simulink model "LoadFlow116BusNetwork_original"  (R2024a)
settings: Solver=FixedStepDiscrete  StartTime=0.0  StopTime=4.5  FixedStep=75e-6  RelTol=1e-3  EnableMultiTasking=on
undefined symbols (not defined in the file or in its folder): D1, D11, Delta
libraries: spsSeriesRLCBranchLib x164, spsLoadFlowBusLib x116, spsDistributedParametersLineLib x79, spsThreePhaseSeriesRLCLoadLib x60, spsThreePhaseTransformerTwoWindingsLib x52, spsThreePhaseParallelRLCLoadLib x44, spsThreePhaseVIMeasurementLib x44, spsSynchronousMachinepuStandardLib x28, spsExcitationSystemLib x28, spsHydraulicTurbineandGovernorLib x28, spsGenericPowerSystemStabilizerLib x28, spsMultiBandPowerSystemStabilizerLib x28
(part 10 of 15)

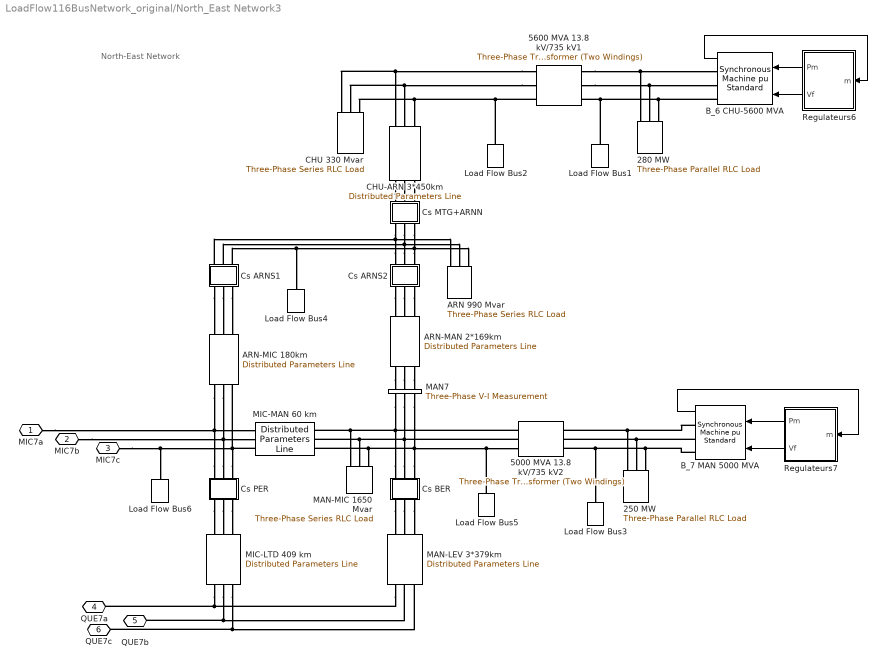
== system LoadFlow116BusNetwork_original/North_East Network3 ==
  note: North-East Network
  250 MW : spsThreePhaseParallelRLCLoadLib/Three-Phase Parallel RLC Load  LConnTagsString=A|B|C  Configuration=Y (grounded)  NominalVoltage=(13800)*1  Vabc=[1e3 1e3 1e3]  Vabcp=[1e3 1e3 1e3]  NominalFrequency=60  UnbalancedPower=off  ActivePower=250000000  InductivePower=0  CapacitivePower=0  Pabc=[10e3 9e3 11e3]  QLabc=[100 90 110]  QCabc=[100 90 110]  Pabcp=[10e3 9e3 11e3]  QLabcp=[100 90 110]  QCabcp=[100 90 110]  Measurements=None  LoadType=constant PQ
  280 MW : spsThreePhaseParallelRLCLoadLib/Three-Phase Parallel RLC Load  LConnTagsString=A|B|C  Configuration=Y (grounded)  NominalVoltage=(13800)*1  Vabc=[1e3 1e3 1e3]  Vabcp=[1e3 1e3 1e3]  NominalFrequency=60  UnbalancedPower=off  ActivePower=280000000  InductivePower=0  CapacitivePower=0  Pabc=[10e3 9e3 11e3]  QLabc=[100 90 110]  QCabc=[100 90 110]  Pabcp=[10e3 9e3 11e3]  QLabcp=[100 90 110]  QCabcp=[100 90 110]  Measurements=None  LoadType=constant PQ
  5000 MVA 13.8 kV/735 kV2 : spsThreePhaseTransformerTwoWindingsLib/Three-Phase Transformer (Two Windings)  Winding1Connection=Delta (D1)  Winding2Connection=Yg  CoreType=Three single-phase transformers  SetSaturation=off  Hysteresis=off  DataFile='basic_model'  SetInitialFlux=off  Measurements=None  UNITS=pu  NominalPower=[ 5000e6 60 ]  Winding1="[ 13.8e3 0.002  0.0]"  Winding2=[ 735e3 0.002 0.12]  Rm=500  Lm=500  L0=0.5  Saturation="[ 0,0  ;  0.005,1.2  ;  1.0,1.4 ]"  InitialFluxes=[ 0.8 , -0.8 , 0.7 ]  BreakLoop=off  DiscreteSolver=Trapezoidal iterative  DataType=off  TransfoNumber=0
  5600 MVA 13.8 kV/735 kV1 : spsThreePhaseTransformerTwoWindingsLib/Three-Phase Transformer (Two Windings)  Winding1Connection=Delta (D1)  Winding2Connection=Yg  CoreType=Three single-phase transformers  SetSaturation=off  Hysteresis=off  DataFile='basic_model'  SetInitialFlux=off  Measurements=None  UNITS=pu  NominalPower=[ 5600e6 60 ]  Winding1="[ 13.8e3 0.002  0.0]"  Winding2=[ 735e3 0.002 0.12]  Rm=500  Lm=500  L0=0.5  Saturation="[ 0,0  ;  0.005,1.2  ;  1.0,1.4 ]"  InitialFluxes=[ 0.8 , -0.8 , 0.7 ]  BreakLoop=off  DiscreteSolver=Trapezoidal iterative  DataType=off  TransfoNumber=0
  ARN 990 Mvar : spsThreePhaseSeriesRLCLoadLib/Three-Phase Series RLC Load  LConnTagsString=A|B|C  Configuration=Y (grounded)  NominalVoltage=735e3  Vabc=[1e3 1e3 1e3]  Vabcp=[1e3 1e3 1e3]  NominalFrequency=60  UnbalancedPower=off  ActivePower=3300000  InductivePower=990e6  CapacitivePower=0  Pabc=[10e3 9e3 11e3]  QLabc=[100 90 110]  QCabc=[100 90 110]  Pabcp=[10e3 9e3 11e3]  QLabcp=[100 90 110]  QCabcp=[100 90 110]  Measurements=None  LoadType=constant Z
  ARN-MAN 2*169km : spsDistributedParametersLineLib/Distributed Parameters Line  Phases=3  Length=169  Frequency=60  Resistance="[0.01273  0.3864]/2"  Inductance="[0.9337e-3  4.1264e-3]/2"  Capacitance=[12.74e-9 7.751e-9]*2  x1=[-0.000975 6.97288339187692e-10 276427.296115167 -784420.047795391;-0.0009 5.9086446365215e-10 298492.841238258 -776291.834335168;-0.000825 4.83968260104895e-10 320319.775751156 -767543.065060241;-0.00075 3.76685179735474e-10 341890.651536376 -758180.733602908;-0.000675 2.69100982996849e-10 363188.22516586 -748212.324067686;-0.0006 1.613016710498e-10 384195.471685113 -737645.805048638;-0.000525 5.33734170149115e-11 404895.598222688 -726489.623259392;-0.00045 -5.45975029128977e-11 425272.057414155 -714752.696780978;-0.000375 -1.62524778432248e-10 445308.560629805 -702444.407932839;-0.0003 -2.70322134130433e-10 464989.090995538 -689574.595772759;-0.000225 -3.7790339845066e-10 484297.9161965 -676153.548231663;-0.00015 -4.85182572576282e-10 503219.601053261 -662191.993889607;-7.5e-05 -5.9207389917693e-10 521739.019860459 -647701.093399513]  x2=[-0.000975 1.79211182163766e-09 170603.864508898 -782532.609847016;-0.0009 1.69187859903041e-09 192658.333570984 -777396.800423744;-0.000825 1.59029291455771e-09 214558.794508984 -771639.551892782;-0.00075 1.48743597426141e-09 236287.740429513 -765265.466510519;-0.000675 1.38339000040582e-09 257827.801545667 -758279.639623281;-0.0006 1.27823816575047e-09 279161.759062162 -750687.655594196;-0.000525 1.17206452706313e-09 300272.558939782 -742495.583339135;-0.00045 1.06495395792605e-09 321143.325528109 -733709.971475316;-0.000375 9.56992080889336e-10 341757.375055666 -724337.843086439;-0.0003 8.48265199025631e-10 362098.228966668 -714386.69010854;-0.000225 7.38860226940719e-10 382149.627093722 -703864.46734105;-0.00015 6.28864621295331e-10 401895.540655962 -692779.586087855;-7.5e-05 5.1836631089363e-10 421320.185072211 -681140.907433425]  x3=[-0.000975 1.85817274928847e-12 1329.17201367229 -2414.87241463209;-0.0009 1.81508564794597e-12 1396.90953145523 -2376.3316706908;-0.000825 1.77054759490824e-12 1463.53038113216 -2335.89132357105;-0.00075 1.72459419321344e-12 1528.98130701517 -2293.58370066758;-0.000675 1.67726217730775e-12 1593.20998863556 -2249.4426220468;-0.0006 1.6285893836805e-12 1656.16508256796 -2203.50337341158;-0.000525 1.57861472061818e-12 1717.79626347353 -2155.80267789439;-0.00045 1.52737813710182e-12 1778.05426432925 -2106.37866670137;-0.000375 1.47492059087233e-12 1836.8909158112 -2055.27084863088;-0.0003 1.42128401568954e-12 1894.25918480043 -2002.52007849068;-0.000225 1.36651128781098e-12 1950.11321198046 -1948.16852443932;-0.00015 1.31064619171726e-12 2004.40834849657 -1892.25963427751;-7.5e-05 1.25373338511145e-12 2057.10119164737 -1834.83810071659]  x4=[-0.000975 2.61332635721004e-12 681.724417841508 -9455.17189861359;-0.0009 2.14673687942227e-12 948.756484622685 -9432.1197918923;-0.000825 1.67843133301927e-12 1215.03012998652 -9401.52779292565;-0.00075 1.20878407428951e-12 1480.33249885502 -9363.42035648953;-0.000675 7.38170532065782e-13 1744.45151257379 -9317.82794508557;-0.0006 2.66966907613108e-13 2007.17603844441 -9264.78700458986;-0.000525 -2.04450126100782e-13 2268.29605850072 -9204.33993511867;-0.00045 -6.75703725512058e-13 2527.60283739395 -9136.53505713448;-0.000375 -1.14641717770377e-12 2784.8890892526 -9061.42657281928;-0.0003 -1.6162142015444e-12 3039.94914338353 -8979.07452274625;-0.000225 -2.08471924848123e-12 3292.57910868201 -8889.54473788418;-0.00015 -2.55155780274809e-12 3542.57703661917 -8792.90878697324;-7.5e-05 -3.01635668074757e-12 3789.7430826765 -8689.24391931401]  x5=0.000955765248222805  V1=ones(3,3)  V2=ones(3,3)  I1=ones(3,3)  I2=ones(3,3)  nHarmo=1  Measurements=None  Decoupling=off  VsMag0=[ 1 1 1]  VrMag0=[ 1 1 1]  VsAngle0=[0 -120 120]  VrAngle0=[0 -120 120]  IsMag0=[ 1 1 1]  IrMag0=[ 1 1 1]  IsAngle0=[0 -120 120]  IrAngle0=[0 -120 120]
      settings: AttributesFormatString=\n  LibrarySourceBlock=sps_lib/Power Grid Elements/Distributed Parameters Line
  ARN-MIC 180km : spsDistributedParametersLineLib/Distributed Parameters Line  Phases=3  Length=180  Frequency=60  Resistance="[0.01273  0.3864]"  Inductance="[0.9337e-3  4.1264e-3]"  Capacitance=[12.74e-9 7.751e-9]  x1=[-0.00105 9.60262409026762e-10 262529.955827452 -774207.772445399;-0.000975 8.43704923918377e-10 284312.349574713 -766476.523484014;-0.0009 7.26472994002931e-10 305867.468379848 -758132.564917239;-0.000825 6.08660332691488e-10 327178.081410689 -749182.566777887;-0.00075 4.90361117622907e-10 348227.153289243 -739633.683557531;-0.000675 3.71669915379674e-10 368997.857709512 -729493.548487313;-0.0006 2.52681605892828e-10 389473.590888184 -718770.26743606;-0.000525 1.33491306596389e-10 409637.984837447 -707472.412430573;-0.00045 1.41942963919424e-11 429474.920449301 -695609.01480328;-0.000375 -1.0511406051586e-10 448968.540380935 -683189.557972727;-0.0003 -2.24338390851985e-10 468103.261730838 -670223.969862682;-0.000225 -3.43383388510955e-10 486863.788495533 -656722.6149659;-0.00015 -4.62153890743092e-10 505235.12379697 -642696.286058906;-7.5e-05 -5.8055495422616e-10 523202.581870801 -628156.195574421]  x2=[-0.00105 3.56382163731829e-09 126759.491965692 -811882.989724104;-0.000975 3.44933874622974e-09 149661.239004238 -807974.954382786;-0.0009 3.3320985065241e-09 172443.349138217 -803421.036225366;-0.000825 3.21219463825516e-09 195087.610697368 -798224.875584341;-0.00075 3.08972299074063e-09 217575.922205467 -792390.626191025;-0.000675 2.96478146594164e-09 239890.306850379 -785922.951855114;-0.0006 2.83746994020147e-09 262012.926854439 -778827.022736515;-0.000525 2.70789018440583e-09 283926.097733704 -771108.511212393;-0.00045 2.5761457826289e-09 305612.302434655 -762773.587342764;-0.000375 2.44234204932968e-09 327054.205337066 -753828.913938241;-0.0003 2.30658594516532e-09 348234.666111827 -744281.641233884;-0.000225 2.16898599148834e-09 369136.753422667 -734139.401173416;-0.00015 2.02965218359636e-09 389743.758460803 -723410.301308359;-7.5e-05 1.88869590280353e-09 410039.208301705 -712102.918316986]  x3=[-0.00105 4.84689301461233e-12 -44.8517351581199 -825.87934362595;-0.000975 4.94622387761714e-12 -21.4861584034094 -826.817643959817;-0.0009 5.04160080493394e-12 1.89659405757936 -827.094998919837;-0.000825 5.13294755370635e-12 25.2778304102975 -826.711186792699;-0.00075 5.22019110274107e-12 48.6388600521494 -825.666514391943;-0.000675 5.30326171087985e-12 71.9610085334751 -823.961816812704;-0.0006 5.38209297274958e-12 95.2256324856196 -821.598456764144;-0.000525 5.45662187184569e-12 118.414134524156 -818.578323480124;-0.00045 5.52678883090655e-12 141.507978115351 -814.903831208983;-0.000375 5.59253775953869e-12 164.488702393985 -810.57791728362;-0.0003 5.65381609905455e-12 187.337936920687 -805.604039773438;-0.000225 5.71057486448711e-12 210.037416366981 -799.986174720016;-0.00015 5.76276868374773e-12 232.568995116311 -793.728812958723;-7.5e-05 5.81035583389588e-12 254.914661769371 -786.836956528808]  x4=[-0.00105 4.98553141097365e-12 787.856966725554 -5164.02437043783;-0.000975 4.55090288137183e-12 933.53262233862 -5139.68710729464;-0.0009 4.11263642963779e-12 1078.46202625692 -5111.24125691772;-0.000825 3.67108239926734e-12 1222.52932413244 -5078.70955848464;-0.00075 3.22659376179636e-12 1365.61935077159 -5042.11801733737;-0.000675 2.77952583464074e-12 1507.6177221964 -5001.49588419404;-0.0006 2.33023599706108e-12 1648.41092708142 -4956.87563176633;-0.000525 1.87908340447918e-12 1787.88641749285 -4908.29292880132;-0.00045 1.42642870137468e-12 1925.93269885773 -4855.78661156844;-0.000375 9.72633732991387e-13 2062.43941909089 -4799.39865281429;-0.0003 5.18061256083737e-13 2197.29745680882 -4739.17412821035;-0.000225 6.30746489345782e-14 2330.39900855955 -4675.16118032011;-0.00015 -3.91962379123865e-13 2461.63767499914 -4607.41098011468;-7.5e-05 -8.46686078453662e-13 2590.90854594566 -4535.97768606751]  x5=0.00101797482059234  V1=ones(3,3)  V2=ones(3,3)  I1=ones(3,3)  I2=ones(3,3)  nHarmo=1  Measurements=None  Decoupling=off  VsMag0=[ 1 1 1]  VrMag0=[ 1 1 1]  VsAngle0=[0 -120 120]  VrAngle0=[0 -120 120]  IsMag0=[ 1 1 1]  IrMag0=[ 1 1 1]  IsAngle0=[0 -120 120]  IrAngle0=[0 -120 120]
      settings: AttributesFormatString=\n  LibrarySourceBlock=sps_lib/Power Grid Elements/Distributed Parameters Line
  "B_6 CHU-5600 MVA " : spsSynchronousMachinepuStandardLib/Synchronous Machine pu Standard  PresetModel=No  MechanicalLoad=Mechanical power Pm  ShowDetailedParameters=on  RotorType=Salient-pole  Units=per unit standard parameters  MeasurementBus=off  NominalParameters="[ 5600E6  13800   60 ]"  Reactances1=[ 31 32 33 34 35 36 37 ]  Reactances2=[ 1.305, 0.296, 0.252, 0.474, 0.243, 0.18 ]  dAxisTimeConstants=Short-circuit  qAxisTimeConstants=Open-circuit  TimeConstants1=[]  TimeConstants2=[]  TimeConstants3=[]  TimeConstants4=[]  TimeConstants5=[ 1.01, 0.053, 0.1 ]  TimeConstants6=[]  TimeConstants7=[]  TimeConstants8=[]  StatorResistance=2.8544e-3  Mechanical="[ 4.0 0  32]"  PolePairs=32  InitialConditions=[0 -61.7964 0.894782 0.894782 0.894782 8.48442 -111.516 128.484 1.31361]  SetSaturation=off  Saturation=[0.6404,0.7127,0.8441,0.9214,0.9956,1.082,1.19,1.316,1.457;0.7,0.7698,0.8872,0.9466,0.9969,1.046,1.1,1.151,1.201]  LoadFlowParameters=[1 5000000000 0 0 0]  TsPowergui=0  TsBlock=-1  IterativeModel=Trapezoidal non iterative  IterativeDiscreteModel=Trapezoidal non iterative  BusType=PV  Pref=5000000000  Qref=0  Qmin=-Inf  Qmax=Inf  PLF=0  QLF=0
  B_7 MAN 5000 MVA : spsSynchronousMachinepuStandardLib/Synchronous Machine pu Standard  PresetModel=No  MechanicalLoad=Mechanical power Pm  ShowDetailedParameters=on  RotorType=Salient-pole  Units=per unit standard parameters  MeasurementBus=off  NominalParameters="[ 5000E6  13800   60 ]"  Reactances1=[ 31 32 33 34 35 36 37 ]  Reactances2=[ 1.305, 0.296, 0.252, 0.474, 0.243, 0.18 ]  dAxisTimeConstants=Short-circuit  qAxisTimeConstants=Open-circuit  TimeConstants1=[]  TimeConstants2=[]  TimeConstants3=[]  TimeConstants4=[]  TimeConstants5=[ 1.01, 0.053, 0.1 ]  TimeConstants6=[]  TimeConstants7=[]  TimeConstants8=[]  StatorResistance=2.8544e-3  Mechanical="[ 3.7 0  32]"  PolePairs=32  InitialConditions=[0 -81.9543 0.907703 0.907703 0.907703 -8.76021 -128.76 111.24 1.25655]  SetSaturation=off  Saturation=[0.6404,0.7127,0.8441,0.9214,0.9956,1.082,1.19,1.316,1.457;0.7,0.7698,0.8872,0.9466,0.9969,1.046,1.1,1.151,1.201]  LoadFlowParameters=[1 4500000000 0 0 0]  TsPowergui=0  TsBlock=-1  IterativeModel=Trapezoidal non iterative  IterativeDiscreteModel=Trapezoidal non iterative  BusType=PV  Pref=4500000000  Qref=0  Qmin=-Inf  Qmax=Inf  PLF=0  QLF=0
  CHU 330 Mvar : spsThreePhaseSeriesRLCLoadLib/Three-Phase Series RLC Load  LConnTagsString=A|B|C  Configuration=Y (grounded)  NominalVoltage=735e3  Vabc=[1e3 1e3 1e3]  Vabcp=[1e3 1e3 1e3]  NominalFrequency=60  UnbalancedPower=off  ActivePower=1100000  InductivePower=330e6  CapacitivePower=0  Pabc=[10e3 9e3 11e3]  QLabc=[100 90 110]  QCabc=[100 90 110]  Pabcp=[10e3 9e3 11e3]  QLabcp=[100 90 110]  QCabcp=[100 90 110]  Measurements=None  LoadType=constant Z
  CHU-ARN 3*450km : spsDistributedParametersLineLib/Distributed Parameters Line  Phases=3  Length=450  Frequency=60  Resistance="[0.01273  0.3864]/3"  Inductance="[0.9337e-3  4.1264e-3]/3"  Capacitance=[12.74e-9 7.751e-9]*3  x1=[-0.00255 1.27916652564422e-09 0 0;-0.002475 1.19821918273683e-09 0 0;-0.0024 1.11631400174812e-09 0 0;-0.002325 1.03351645642659e-09 0 0;-0.00225 9.4989273386313e-10 0 0;-0.002175 8.65509681582063e-10 0 0;-0.0021 7.80434754104282e-10 0 0;-0.002025 6.94735959025121e-10 0 0;-0.00195 6.08481802650133e-10 0 0;-0.001875 5.2174123523219e-10 0 0;-0.0018 4.34583595853711e-10 0 0;-0.001725 3.47078556998058e-10 0 0;-0.00165 2.59296068854421e-10 0 0;-0.001575 1.71306303400705e-10 242668.421457094 -732167.508894252;-0.0015 8.31795983091243e-11 263270.288908761 -725014.590467024;-0.001425 -5.01359928065404e-12 283661.702119646 -717282.106469271;-0.00135 -9.32027890758778e-11 303826.360506025 -708976.23813039;-0.001275 -1.81317473987565e-10 323748.144748515 -700103.625034449;-0.0012 -2.69287216484797e-10 343411.129677606 -690671.359812599;-0.001125 -3.57041694901403e-10 362799.597003999 -680686.982473342;-0.00105 -4.44510759650027e-10 381898.047883567 -670158.474375156;-0.000975 -5.31624489298628e-10 400691.215306893 -659094.251846322;-0.0009 -6.18313246464612e-10 419164.076303483 -647503.159457043;-0.000825 -7.04507733481883e-10 437301.863950903 -635394.462949224;-0.00075 -7.90139047796337e-10 455090.079179222 -622777.841829585;-0.000675 -8.75138737045516e-10 472514.502361358 -609663.381632008;-0.0006 -9.59438853778372e-10 489561.20468002 -596061.565855317;-0.000525 -1.04297200977143e-09 506216.559262199 -581983.267582929;-0.00045 -1.12567142989787e-09 522467.252072276 -567439.740791078;-0.000375 -1.20747100550661e-09 538300.292555064 -552442.611352557;-0.0003 -1.28830534726847e-09 553703.024020254 -537003.867743177;-0.000225 -1.36810983744746e-09 568663.133759983 -521135.851458357;-0.00015 -1.44682068155518e-09 583168.662891422 -504851.247147528;-7.5e-05 -1.52437495934716e-09 597208.015916525 -488163.072474212]  x2=[-0.00255 2.8073590882473e-09 0 0;-0.002475 2.72875365746816e-09 0 0;-0.0024 2.64796690276658e-09 0 0;-0.002325 2.56506340383818e-09 0 0;-0.00225 2.48010943247153e-09 0 0;-0.002175 2.39317289957151e-09 0 0;-0.0021 2.30432330087236e-09 0 0;-0.002025 2.21363166138381e-09 0 0;-0.00195 2.12117047861485e-09 0 0;-0.001875 2.02701366462028e-09 0 0;-0.0018 1.93123648691657e-09 0 0;-0.001725 1.83391550831412e-09 0 0;-0.00165 1.73512852571417e-09 0 0;-0.001575 1.63495450791913e-09 -54170.2857366766 -807523.190587066;-0.0015 1.5334735325061e-09 -31319.4766466056 -808731.868853668;-0.001425 1.43076672181411e-09 -8443.63124610734 -809294.059238321;-0.00135 1.32691617809617e-09 14438.9638640172 -809209.312334633;-0.001275 1.22200491788796e-09 37310.0166873523 -808477.695887982;-0.0012 1.11611680564569e-09 60151.24445421 -807099.794741363;-0.001125 1.00933648670615e-09 82944.3882365959 -805076.710367868;-0.00105 9.01749319622503e-10 105671.227544117 -802410.059990191;-0.000975 7.93441307929975e-10 128313.594889164 -799101.975287844;-0.0009 6.84499031395948e-10 150853.39030972 -795155.100693122;-0.000825 5.75009576809409e-10 173272.595838196 -790572.591277188;-0.00075 4.65060468365111e-10 195553.289904719 -785358.110227952;-0.000675 3.54739597698064e-10 217677.661663358 -779515.825921782;-0.0006 2.44135153624316e-10 239628.025229844 -773050.408591363;-0.000525 1.33335551644154e-10 261386.833819392 -765967.026592383;-0.00045 2.24293632641098e-11 282936.693773338 -758271.342272034;-0.000375 -8.84947548057469e-11 304260.378463357 -749969.507442613;-0.0003 -1.99348131522627e-10 325340.842062174 -741068.158463861;-0.000225 -3.10042152393297e-10 346161.233169727 -731574.410937956;-0.00015 -4.20488330311147e-10 366704.908283929 -721495.854021411;-7.5e-05 -5.30598376291434e-10 386955.445105222 -710840.544358418]  x3=[-0.00255 8.71375892097744e-12 0 0;-0.002475 8.68441234844256e-12 0 0;-0.0024 8.6481235895523e-12 0 0;-0.002325 8.60492165298529e-12 0 0;-0.00225 8.55484107370859e-12 0 0;-0.002175 8.49792188537102e-12 0 0;-0.0021 8.43420958830086e-12 0 0;-0.002025 8.36375511313354e-12 0 0;-0.00195 8.28661478009853e-12 0 0;-0.001875 8.20285025399776e-12 0 0;-0.0018 8.11252849491177e-12 0 0;-0.001725 8.01572170467279e-12 0 0;-0.00165 7.91250726914775e-12 0 0;-0.001575 7.80296769637718e-12 -1464.09976004949 -2947.40439174756;-0.0015 7.68719055061953e-12 -1380.1903706523 -2987.61903902201;-0.001425 7.56526838235368e-12 -1295.17767819044 -3025.44542934877;-0.00135 7.43729865429546e-12 -1209.12964050951 -3060.85332489018;-0.001275 7.30338366348748e-12 -1122.11504309426 -3093.8144211163;-0.0012 7.16363045952442e-12 -1034.2034440825 -3124.30236943112;-0.001125 7.01815075897925e-12 -945.465118661389 -3152.29279823525;-0.00105 6.86706085609865e-12 -855.971002890517 -3177.76333240817;-0.000975 6.71048152983925e-12 -765.792636996729 -3200.69361119457;-0.0009 6.5485379473187e-12 -675.002108185947 -3221.06530448044;-0.000825 6.38135956375905e-12 -583.671993017759 -3238.86212744585;-0.00075 6.20908001900221e-12 -491.875299388834 -3254.06985358284;-0.000675 6.03183703068029e-12 -399.685408171522 -3266.67632606781;-0.0006 5.84977228412625e-12 -307.17601455431 -3276.67146747955;-0.000525 5.66303131911279e-12 -214.421069131013 -3284.04728785494;-0.00045 5.47176341351012e-12 -121.494718785806 -3288.79789107603;-0.000375 5.27612146395547e-12 -28.4712474213323 -3290.91947958328;-0.0003 5.07626186362991e-12 64.574983422705 -3290.41035741132;-0.000225 4.87234437723997e-12 157.569594013025 -3287.2709315446;-0.00015 4.66453201330424e-12 250.438245880786 -3281.50371159214;-7.5e-05 4.4529908938468e-12 343.106701246624 -3273.11330778133]  x4=[-0.00255 1.41679352076083e-11 0 0;-0.002475 1.37991525490882e-11 0 0;-0.0024 1.34193390591544e-11 0 0;-0.002325 1.30287983548995e-11 0 0;-0.00225 1.2627842628587e-11 0 0;-0.002175 1.22167923980897e-11 0 0;-0.0021 1.17959762506726e-11 0 0;-0.002025 1.13657305803251e-11 0 0;-0.00195 1.09263993188533e-11 0 0;-0.001875 1.04783336609455e-11 0 0;-0.0018 1.0021891783433e-11 0 0;-0.001725 9.55743855896888e-12 0 0;-0.00165 9.08534526435446e-12 0 0;-0.001575 8.60598928374616e-12 -1565.83540458993 -14460.8260986629;-0.0015 8.11975380698048e-12 -1156.39187005692 -14499.3124213111;-0.001425 7.62702752325791e-12 -746.023933556372 -14526.2082154565;-0.00135 7.12820431043067e-12 -335.059636937891 -14541.4919810129;-0.001275 6.62368292014287e-12 76.172501227773 -14545.151500372;-0.0012 6.11386665907444e-12 487.343748261434 -14537.18384817;-0.001125 5.59916306654405e-12 898.125420159345 -14517.5953936261;-0.00105 5.07998358872833e-12 1308.18914433816 -14486.4017954513;-0.000975 4.55674324975814e-12 1717.20712213096 -14443.6279893305;-0.0009 4.0298603199546e-12 2124.85239082447 -14389.30816799;-0.000825 3.49975598147022e-12 2530.79908502809 -14323.4857538637;-0.00075 2.96685399160232e-12 2934.72269716567 -14246.2133643825;-0.000675 2.43158034404791e-12 3336.30033688189 -14157.5527699123;-0.0006 1.8943629283709e-12 3735.21098915592 -14057.5748443755;-0.000525 1.35563118795368e-12 4131.13577091586 -13946.3595085963;-0.00045 8.15815776706656e-13 4523.75818594903 -13823.9956664123;-0.000375 2.75348214810135e-13 4912.76437790417 -13690.5811336069;-0.0003 -2.65339456236336e-13 5297.84338118343 -13546.2225597162;-0.000225 -8.05815018981322e-13 5678.68736952349 -13391.0353427753;-0.00015 -1.34564642552952e-12 6054.99190206719 -13225.1435370712;-7.5e-05 -1.88440214291423e-12 6426.45616672885 -13048.679753975]  x5=0.00254493705148084  V1=ones(3,3)  V2=ones(3,3)  I1=ones(3,3)  I2=ones(3,3)  nHarmo=1  Measurements=None  Decoupling=off  VsMag0=[ 1 1 1]  VrMag0=[ 1 1 1]  VsAngle0=[0 -120 120]  VrAngle0=[0 -120 120]  IsMag0=[ 1 1 1]  IrMag0=[ 1 1 1]  IsAngle0=[0 -120 120]  IrAngle0=[0 -120 120]
      settings: AttributesFormatString=\n  LibrarySourceBlock=sps_lib/Power Grid Elements/Distributed Parameters Line
  "Cs ARNS1 " : Subsystem  mask{Xc=25}
      mask prompts: Xc "Condensator Reactance at  60Hz  (ohm):"
      mask help: Series Compensation
      mask init:
      | Cs=1/Xc/(2*pi*60);
      mask Display: disp('Cs')
  Cs ARNS2 : Subsystem  mask{Xc=25/2}
      mask prompts: Xc "Condensator Reactance at  60Hz  (ohm):"
      mask help: Series Compensation
      mask init:
      | Cs=1/Xc/(2*pi*60);
      mask Display: disp('Cs')
  Cs BER : Subsystem  mask{Xc=22/3}
      mask prompts: Xc "Condensator Reactance at  60Hz  (ohm):"
      mask help: Series Compensation
      mask init:
      | Cs=1/Xc/(2*pi*60);
      mask Display: disp('Cs')
  "Cs MTG+ARNN " : Subsystem  mask{Xc=(30+25)/3}
      mask prompts: Xc "Condensator Reactance at  60Hz  (ohm):"
      mask help: Series Compensation
      mask init:
      | Cs=1/Xc/(2*pi*60);
      mask Display: disp('Cs')
  "Cs PER " : Subsystem  mask{Xc=22}
      mask prompts: Xc "Condensator Reactance at  60Hz  (ohm):"
      mask help: Series Compensation
      mask init:
      | Cs=1/Xc/(2*pi*60);
      mask Display: disp('Cs')
  Load Flow Bus1 : spsLoadFlowBusLib/Load Flow Bus  LConnTagsString=a  Phases=single  Connectors=on one side  ID=CHU_13.8  Vbase=13.8e3  Vref=1  Vangle=0  VLF=1  VLFb=1  VLFc=1  angleLF=4.726  angleLFb=0  angleLFc=0
      settings: AttributesFormatString=%<ID>\n%<Vbase>V\n%<VLF>pu\n%<angleLF>deg.
  Load Flow Bus2 : spsLoadFlowBusLib/Load Flow Bus  LConnTagsString=a  Phases=single  Connectors=on one side  ID=CHU7  Vbase=735e3  Vref=1  Vangle=0  VLF=1.009  VLFb=1  VLFc=1  angleLF=28.97  angleLFb=0  angleLFc=0
      settings: AttributesFormatString=%<ID>\n%<Vbase>V\n%<VLF>pu\n%<angleLF>deg.
  Load Flow Bus3 : spsLoadFlowBusLib/Load Flow Bus  LConnTagsString=a  Phases=single  Connectors=on one side  ID=MAN_13.8  Vbase=13.8e3  Vref=1  Vangle=0  VLF=1  VLFb=1  VLFc=1  angleLF=-16.23  angleLFb=0  angleLFc=0
      settings: AttributesFormatString=%<ID>\n%<Vbase>V\n%<VLF>pu\n%<angleLF>deg.
  Load Flow Bus4 : spsLoadFlowBusLib/Load Flow Bus  LConnTagsString=a  Phases=single  Connectors=on one side  ID=ARN7  Vbase=735e3  Vref=1  Vangle=0  VLF=1.054  VLFb=1  VLFc=1  angleLF=12.72  angleLFb=0  angleLFc=0
      settings: AttributesFormatString=%<ID>\n%<Vbase>V\n%<VLF>pu\n%<angleLF>deg.
  Load Flow Bus5 : spsLoadFlowBusLib/Load Flow Bus  LConnTagsString=a  Phases=single  Connectors=on one side  ID=MAN7  Vbase=735e3  Vref=1  Vangle=0  VLF=1.016  VLFb=1  VLFc=1  angleLF=7.996  angleLFb=0  angleLFc=0
      settings: AttributesFormatString=%<ID>\n%<Vbase>V\n%<VLF>pu\n%<angleLF>deg.
  Load Flow Bus6 : spsLoadFlowBusLib/Load Flow Bus  LConnTagsString=a  Phases=single  Connectors=on one side  ID=MIC7  Vbase=735e3  Vref=1  Vangle=0  VLF=1.041  VLFb=1  VLFc=1  angleLF=5.981  angleLFb=0  angleLFc=0
      settings: AttributesFormatString=%<ID>\n%<Vbase>V\n%<VLF>pu\n%<angleLF>deg.
  MAN-LEV 3*379km : spsDistributedParametersLineLib/Distributed Parameters Line  Phases=3  Length=379  Frequency=60  Resistance="[0.01273  0.3864]/3"  Inductance="[0.9337e-3  4.1264e-3]/3"  Capacitance=[12.74e-9 7.751e-9]*3  x1=[-0.002175 2.13330351564683e-09 -129715.856576042 -778750.814672818;-0.0021 2.13919297136545e-09 -107648.251269204 -782106.718665322;-0.002025 2.1433723889535e-09 -85494.5935973747 -784837.418513559;-0.00195 2.14583842744853e-09 -63272.5928555347 -786940.731337852;-0.001875 2.14658911553708e-09 -41000.0129710692 -788414.975782109;-0.0018 2.14562385313058e-09 -18694.6583035559 -789258.973357881;-0.001725 2.14294341184504e-09 3625.64058776759 -789472.049386417;-0.00165 2.13854993438421e-09 25943.0411974792 -789054.033538001;-0.001575 2.13244693282674e-09 48239.7033369995 -788005.259968107;-0.0015 2.12463928581869e-09 70497.8033957643 -786326.567050279;-0.001425 2.11513323467364e-09 92699.5485891471 -784019.29670595;-0.00135 2.10393637838341e-09 114827.191181738 -781085.293331733;-0.001275 2.09105766754361e-09 136863.042674614 -777526.902325032;-0.0012 2.07650739719863e-09 158789.48794525 -773346.968209172;-0.001125 2.06029719861196e-09 180588.999328784 -768548.832359532;-0.00105 2.04244002996832e-09 202244.150629358 -763136.330332495;-0.000975 2.0229501660151e-09 223737.631050359 -757113.788799368;-0.0009 2.00184318665135e-09 245052.259032398 -750486.022087704;-0.000825 1.97913596447342e-09 266170.995987993 -743258.328332804;-0.00075 1.95484665128728e-09 287076.959921947 -735436.485242468;-0.000675 1.92899466359826e-09 307753.438926564 -727026.745478386;-0.0006 1.90160066708977e-09 328183.904540889 -718035.83165785;-0.000525 1.87268656010347e-09 348352.024963306 -708470.930979803;-0.00045 1.84227545613409e-09 368241.678106933 -698339.6894795;-0.000375 1.81039166535283e-09 387836.964487367 -687650.205916383;-0.0003 1.77706067517422e-09 407122.219932494 -676411.025300057;-0.000225 1.74230912988181e-09 426082.028104187 -664631.132059542;-0.00015 1.7061648093292e-09 444701.232821886 -652319.942861256;-7.5e-05 1.6686566067332e-09 462964.950178225 -639487.299081476]  x2=[-0.002175 7.58506762929816e-09 -453830.168532003 -672756.853007217;-0.0021 7.58450099144082e-09 -434629.546160044 -685317.991887075;-0.002025 7.57787141953768e-09 -415081.48757894 -697331.298049935;-0.00195 7.56518421316708e-09 -395201.619207625 -708787.16824266;-0.001875 7.54644951428768e-09 -375005.832708703 -719676.4448179;-0.0018 7.5216822991311e-09 -354510.272284895 -729990.423054571;-0.001725 7.4909023662302e-09 -333731.321773612 -739720.85811628;-0.00165 7.45413432059238e-09 -312685.591549964 -748859.97164212;-0.001575 7.41140755403076e-09 -291389.90524868 -757400.45796457;-0.0015 7.36275622166878e-09 -269861.286315556 -765335.48994954;-0.001425 7.30821921463715e-09 -248116.944399167 -772658.72445387;-0.00135 7.24784012898485e-09 -226174.261593741 -779364.307395946;-0.001275 7.1816672308291e-09 -204050.778544181 -785446.878435363;-0.0012 7.10975341777223e-09 -181764.180424333 -790901.575257899;-0.001125 7.03215617661606e-09 -159332.28279974 -795724.037462375;-0.00105 6.94893753740791e-09 -136773.017386142 -799910.410046289;-0.000975 6.86016402385466e-09 -114104.417715143 -803457.346487451;-0.0009 6.76590660014477e-09 -91344.6047184784 -806362.011419141;-0.000825 6.66624061422056e-09 -68511.7722424214 -808622.082896655;-0.00075 6.56124573754625e-09 -45624.1725038991 -810235.754253435;-0.000675 6.45100590141978e-09 -22700.1014999503 -811201.735545287;-0.0006 6.3356092298794e-09 242.115617814212 -811519.254581546;-0.000525 6.21514796925874e-09 23184.1391920584 -811188.057542354;-0.00045 6.0897184144464e-09 46107.6297201617 -810208.409181557;-0.000375 5.95942083190936e-09 68994.262514537 -808581.092615064;-0.0003 5.8243593795415e-09 91825.7423511058 -806307.40869484;-0.000225 5.68464202340132e-09 114583.81809422 -803389.174969022;-0.00015 5.54038045140557e-09 137250.297286341 -799828.724229001;-7.5e-05 5.39168998404763e-09 159807.060690812 -795628.902644621]  x3=[-0.002175 1.48108531847404e-11 -1369.21748804057 -554.792265211392;-0.0021 1.56030075517418e-11 -1352.98611910076 -593.279680632587;-0.002025 1.63826891132403e-11 -1335.67319375873 -631.292837354568;-0.00195 1.71492746037253e-11 -1317.29255170209 -668.801348241473;-0.001875 1.79021512264847e-11 -1297.85888613487 -705.775229563596;-0.0018 1.86407171434658e-11 -1277.38773203198 -742.18492496593;-0.001725 1.9364381956375e-11 -1255.8954537208 -778.001329095056;-0.00165 2.00725671786332e-11 -1233.39923179975 -813.195810865523;-0.001575 2.07647066978093e-11 -1209.91704940445 -847.740236347097;-0.0015 2.14402472281619e-11 -1185.4676778322 -881.606991254596;-0.001425 2.20986487529271e-11 -1160.07066153656 -914.769003022326;-0.00135 2.27393849559999e-11 -1133.74630250376 -947.199762445474;-0.001275 2.33619436426631e-11 -1106.51564402364 -978.873344871166;-0.0012 2.39658271490281e-11 -1078.40045386794 -1009.76443092223;-0.001125 2.45505527398596e-11 -1049.4232068895 -1039.84832673713;-0.00105 2.51156529944669e-11 -1019.60706705619 -1069.10098370985;-0.000975 2.56606761803528e-11 -988.975868933988 -1097.49901771399;-0.0009 2.61851866143216e-11 -957.554098633996 -1125.01972779566;-0.000825 2.66887650107578e-11 -925.366874238624 -1151.64111432032;-0.00075 2.71710088167961e-11 -892.439925722575 -1177.34189655888;-0.000675 2.76315325341167e-11 -858.799574384691 -1202.10152969927;-0.0006 2.80699680271061e-11 -824.472711807118 -1225.90022126959;-0.000525 2.84859648171396e-11 -789.486778358582 -1248.71894695993;-0.00045 2.88791903627481e-11 -753.86974125898 -1270.53946583011;-0.000375 2.92493303254471e-11 -717.650072222808 -1291.34433489121;-0.0003 2.95960888210137e-11 -680.856724699316 -1311.11692304923;-0.000225 2.99191886560121e-11 -643.519110727556 -1329.84142439973;-0.00015 3.02183715493778e-11 -605.667077424854 -1347.50287086281;-7.5e-05 3.04933983388835e-11 -567.330883127475 -1364.08714414842]  x4=[-0.002175 2.16802957646551e-11 -9019.3501694102 -13700.3757737262;-0.0021 2.11951006451567e-11 -8628.42708034702 -13949.8814959029;-0.002025 2.06929624864986e-11 -8230.60655869516 -14188.2358962521;-0.00195 2.01742826902416e-11 -7826.2066160928 -14415.2484379131;-0.001875 1.9639475881079e-11 -7415.5505236665 -14630.7376505335;-0.0018 1.90889695753911e-11 -6998.96655361332 -14834.5312753339;-0.001725 1.85232038394957e-11 -6576.78771678495 -15026.4664028087;-0.00165 1.79426309378655e-11 -6149.35149648401 -15206.3896029538;-0.001575 1.7347714971595e-11 -5716.99957868502 -15374.1570479159;-0.0015 1.67389315074052e-11 -5280.07757889585 -15529.6346269663;-0.001425 1.61167671974825e-11 -4838.93476587801 -15672.6980537073;-0.00135 1.54817193904571e-11 -4393.92378244651 -15803.2329654245;-0.001275 1.48342957338291e-11 -3945.40036357261 -15921.1350145067;-0.0012 1.41750137681639e-11 -3493.72305201472 -16026.3099518598;-0.001125 1.35044005133773e-11 -3039.25291170481 -16118.6737022482;-0.00105 1.28229920474447e-11 -2582.3532391194 -16198.152431503;-0.000975 1.21313330778676e-11 -2123.38927286598 -16264.6826055441;-0.0009 1.14299765062438e-11 -1662.72790171677 -16318.2110411683;-0.000825 1.07194829862853e-11 -1200.73737132352 -16358.6949485632;-0.00075 1.00004204756412e-11 -737.786989847531 -16386.1019655127;-0.000675 9.27336378188047e-12 -274.246832740377 -16400.4101832666;-0.0006 8.5388941029997e-12 189.512553088751 -16401.6081640548;-0.000525 7.79759856282245e-12 653.12044548258 -16389.6949502296;-0.00045 7.05006974166134e-12 1116.20624338537 -16364.680065032;-0.000375 6.29690520261843e-12 1578.39976309572 -16326.5835049784;-0.0003 5.53870701390243e-12 2039.33153418578 -16275.435723876;-0.000225 4.77608126754457e-12 2498.63309485024 -16211.2776084785;-0.00015 4.00963759489794e-12 2955.93728644903 -16134.1604458016;-7.5e-05 3.23998867930745e-12 3410.8785470084 -16044.1458821253]  x5=0.00214340253891386  V1=ones(3,3)  V2=ones(3,3)  I1=ones(3,3)  I2=ones(3,3)  nHarmo=1  Measurements=None  Decoupling=off  VsMag0=[ 1 1 1]  VrMag0=[ 1 1 1]  VsAngle0=[0 -120 120]  VrAngle0=[0 -120 120]  IsMag0=[ 1 1 1]  IrMag0=[ 1 1 1]  IsAngle0=[0 -120 120]  IrAngle0=[0 -120 120]
      settings: AttributesFormatString=\n  LibrarySourceBlock=sps_lib/Power Grid Elements/Distributed Parameters Line
  MAN-MIC 1650 Mvar : spsThreePhaseSeriesRLCLoadLib/Three-Phase Series RLC Load  LConnTagsString=A|B|C  Configuration=Y (grounded)  NominalVoltage=735e3  Vabc=[1e3 1e3 1e3]  Vabcp=[1e3 1e3 1e3]  NominalFrequency=60  UnbalancedPower=off  ActivePower=5500000  InductivePower=1650e6  CapacitivePower=0  Pabc=[10e3 9e3 11e3]  QLabc=[100 90 110]  QCabc=[100 90 110]  Pabcp=[10e3 9e3 11e3]  QLabcp=[100 90 110]  QCabcp=[100 90 110]  Measurements=None  LoadType=constant Z
  MAN7 : spsThreePhaseVIMeasurementLib/Three-Phase V-I Measurement  VoltageMeasurement=no  SetLabelV=on  LabelV=Vabc_MAN7  Vpu=on  VpuLL=off  CurrentMeasurement=no  SetLabelI=on  LabelI=Iabc_MAN7  Ipu=on  Pbase=100e6  Vbase=735e3  OutputType=Magnitude  PhasorSimulation=off  PSBequivalent=0
  MIC-LTD 409 km : spsDistributedParametersLineLib/Distributed Parameters Line  Phases=3  Length=409  Frequency=60  Resistance="[0.01273  0.3864]"  Inductance="[0.9337e-3  4.1264e-3]"  Capacitance=[12.74e-9 7.751e-9]  x1=[-0.002325 3.71222948841858e-09 0 0;-0.00225 3.6619118362838e-09 0 0;-0.002175 3.60866690785623e-09 0 0;-0.0021 3.55253726631698e-09 0 0;-0.002025 3.49356778084267e-09 0 0;-0.00195 3.43180559073774e-09 0 0;-0.001875 3.36730006775196e-09 0 0;-0.0018 3.30010277661344e-09 0 0;-0.001725 3.23026743380856e-09 0 0;-0.00165 3.15784986464184e-09 0 0;-0.001575 3.08290795861005e-09 0 0;-0.0015 3.00550162312622e-09 0 0;-0.001425 2.92569273563057e-09 59193.0163103363 -807702.943453704;-0.00135 2.84354509412667e-09 82003.6023342905 -805706.722468891;-0.001275 2.75912436618222e-09 104748.635933236 -803066.431857862;-0.0012 2.67249803643546e-09 127409.935075324 -799784.182228534;-0.001125 2.58373535264897e-09 149969.38466475 -795862.597361042;-0.00105 2.49290727035405e-09 172408.951022684 -791304.812110325;-0.000975 2.40008639612996e-09 194710.696303116 -786114.469900176;-0.0009 2.30534692956336e-09 216856.792832096 -780295.719810745;-0.000825 2.20876460393426e-09 238829.537358907 -773853.213261821;-0.00075 2.11041662567601e-09 260611.365207768 -766792.100294567;-0.000675 2.01038161265765e-09 282184.864318769 -759118.02545465;-0.0006 1.908739531338e-09 303532.789166806 -750837.12328008;-0.000525 1.80557163284169e-09 324638.074547392 -741956.013397353;-0.00045 1.70096038800826e-09 345483.849218313 -732481.795229824;-0.000375 1.59498942146623e-09 366053.449386249 -722422.042322536;-0.0003 1.48774344478483e-09 386330.432027552 -711784.796288042;-0.000225 1.37930818875691e-09 406298.588032545 -700578.560378069;-0.00015 1.26977033486702e-09 425941.955162842 -688812.292686141;-7.5e-05 1.15921744599957e-09 445244.830811313 -676495.398986621]  x2=[-0.002325 7.58299376641166e-09 0 0;-0.00225 7.58990846809542e-09 0 0;-0.002175 7.59075591307927e-09 0 0;-0.0021 7.58553542392867e-09 0 0;-0.002025 7.57425117382276e-09 0 0;-0.00195 7.55691218321842e-09 0 0;-0.001875 7.53353231263946e-09 0 0;-0.0018 7.50413025159668e-09 0 0;-0.001725 7.46872950364782e-09 0 0;-0.00165 7.42735836760913e-09 0 0;-0.001575 7.38004991493378e-09 0 0;-0.0015 7.32684196327497e-09 0 0;-0.001425 7.26777704625516e-09 -248116.944399167 -772658.724453869;-0.00135 7.2029023794653e-09 -226174.261593742 -779364.307395945;-0.001275 7.13226982272139e-09 -204050.778544181 -785446.878435363;-0.0012 7.05593583860859e-09 -181764.180424333 -790901.575257899;-0.001125 6.97396144734584e-09 -159332.28279974 -795724.037462375;-0.00105 6.88641217800728e-09 -136773.017386142 -799910.410046289;-0.000975 6.79335801613925e-09 -114104.417715143 -803457.346487451;-0.0009 6.69487334781498e-09 -91344.6047184787 -806362.011419141;-0.000825 6.59103690017147e-09 -68511.7722424217 -808622.082896655;-0.00075 6.48193167847621e-09 -45624.1725038994 -810235.754253435;-0.000675 6.36764489977405e-09 -22700.1014999507 -811201.735545287;-0.0006 6.24826792316725e-09 242.115617813834 -811519.254581546;-0.000525 6.12389617678437e-09 23184.139192058 -811188.057542354;-0.00045 5.99462908149653e-09 46107.6297201613 -810208.409181557;-0.000375 5.86056997144184e-09 68994.2625145366 -808581.092615064;-0.0003 5.7218260114217e-09 91825.7423511055 -806307.40869484;-0.000225 5.57850811123491e-09 114583.81809422 -803389.174969022;-0.00015 5.43073083701803e-09 137250.297286341 -799828.724229001;-7.5e-05 5.27861231966301e-09 159807.060690811 -795628.902644621]  x3=[-0.002325 3.31134896168016e-12 0 0;-0.00225 3.4872527829871e-12 0 0;-0.002175 3.66036894777607e-12 0 0;-0.0021 3.83055906963371e-12 0 0;-0.002025 3.9976871011806e-12 0 0;-0.00195 4.16161944282548e-12 0 0;-0.001875 4.32222504956267e-12 0 0;-0.0018 4.4793755357275e-12 0 0;-0.001725 4.63294527762582e-12 0 0;-0.00165 4.78281151395564e-12 0 0;-0.001575 4.92885444394068e-12 0 0;-0.0015 5.07095732309723e-12 0 0;-0.001425 5.20900655655795e-12 -412.085781584141 -775.71082951457;-0.00135 5.34289178987783e-12 -389.991383899217 -787.050857737797;-0.001275 5.47250599724986e-12 -367.585233069073 -797.761729547631;-0.0012 5.59774556705984e-12 -344.885240227856 -807.834882837028;-0.001125 5.7185103847119e-12 -321.909551402522 -817.262265281373;-0.00105 5.83470391265856e-12 -298.676533007178 -826.036340775385;-0.000975 5.9462332675714e-12 -275.204757161253 -834.15009545736;-0.0009 6.05300929459057e-12 -251.512986843227 -841.597043315952;-0.000825 6.15494663859379e-12 -227.620160891795 -848.371231374983;-0.00075 6.25196381242795e-12 -203.545378866453 -854.467244452168;-0.000675 6.34398326204872e-12 -179.307885779593 -859.880209487925;-0.0006 6.43093142851601e-12 -154.927056712344 -864.605799440826;-0.000525 6.51273880679589e-12 -130.422381326422 -868.640236746566;-0.00045 6.58934000132186e-12 -105.813448284397 -871.980296337693;-0.000375 6.66067377827106e-12 -81.119929590814 -874.623308221673;-0.0003 6.72668311451363e-12 -56.3615648666924 -876.567159615246;-0.000225 6.78731524319617e-12 -31.5581455699773 -877.810296633349;-0.00015 6.8425216959227e-12 -6.7294991745493 -878.351725531272;-7.5e-05 6.8922583414996e-12 18.104526679554 -878.191013499038]  x4=[-0.002325 1.04493439585022e-11 0 0;-0.00225 1.03943451580949e-11 0 0;-0.002175 1.03310372772071e-11 0 0;-0.0021 1.02594709231901e-11 0 0;-0.002025 1.01797033050922e-11 0 0;-0.00195 1.00917981879269e-11 0 0;-0.001875 9.99582584169993e-12 0 0;-0.0018 9.89186298523632e-12 0 0;-0.001725 9.7799927248529e-12 0 0;-0.00165 9.66030448792414e-12 0 0;-0.001575 9.53289395139534e-12 0 0;-0.0015 9.39786296529997e-12 0 0;-0.001425 9.25531947134226e-12 -1850.18013712909 -4788.09574636232;-0.00135 9.1053774166103e-12 -1714.07818949483 -4838.48753312468;-0.001275 8.94815666248844e-12 -1576.60603398217 -4885.0115069844;-0.0012 8.78378288884198e-12 -1437.87356372882 -4927.63047738862;-0.001125 8.61238749355057e-12 -1297.99167934882 -4966.3103753845;-0.00105 8.43410748747076e-12 -1157.0722002803 -5001.02028085338;-0.000975 8.24908538491163e-12 -1015.22777539867 -5031.73244722793;-0.0009 8.05746908971105e-12 -872.57179296689 -5058.42232367226;-0.000825 7.85941177700356e-12 -729.21828999461 -5081.06857470749;-0.00075 7.65507177077457e-12 -585.281861078723 -5099.65309726707;-0.000675 7.44461241729855e-12 -440.877566798201 -5114.16103516799;-0.0006 7.22820195456252e-12 -296.120841736435 -5124.58079098669;-0.000525 7.00601337777922e-12 -151.127402204585 -5130.90403532979;-0.00045 6.77822430109733e-12 -6.01315373973944 -5133.12571349252;-0.000375 6.54501681561944e-12 139.105901548201 -5131.24404949933;-0.0003 6.30657734384127e-12 284.113757706836 -5125.26054752364;-0.000225 6.06309649062829e-12 428.894497674646 -5115.17999068537;-0.00015 5.8147688908492e-12 573.332385943321 -5101.01043722744;-7.5e-05 5.5617930537877e-12 717.311961074952 -5082.76321407405]  x5=0.00231306500901259  V1=ones(3,3)  V2=ones(3,3)  I1=ones(3,3)  I2=ones(3,3)  nHarmo=1  Measurements=None  Decoupling=off  VsMag0=[ 1 1 1]  VrMag0=[ 1 1 1]  VsAngle0=[0 -120 120]  VrAngle0=[0 -120 120]  IsMag0=[ 1 1 1]  IrMag0=[ 1 1 1]  IsAngle0=[0 -120 120]  IrAngle0=[0 -120 120]
      settings: AttributesFormatString=\n  LibrarySourceBlock=sps_lib/Power Grid Elements/Distributed Parameters Line
  MIC-MAN 60 km : spsDistributedParametersLineLib/Distributed Parameters Line  Phases=3  Length=60  Frequency=60  Resistance="[0.01273  0.3864]"  Inductance="[0.9337e-3  4.1264e-3]"  Capacitance=[12.74e-9 7.751e-9]  x1=[-0.000375 2.44234204932968e-09 327054.205337066 -753828.913938241;-0.0003 2.30658594516532e-09 348234.666111827 -744281.641233884;-0.000225 2.16898599148834e-09 369136.753422667 -734139.401173416;-0.00015 2.02965218359636e-09 389743.758460803 -723410.301308359;-7.5e-05 1.88869590280353e-09 410039.208301705 -712102.918316986]  x2=[-0.000375 9.56992080889336e-10 341757.375055666 -724337.843086439;-0.0003 8.48265199025631e-10 362098.228966668 -714386.69010854;-0.000225 7.38860226940719e-10 382149.627093722 -703864.46734105;-0.00015 6.28864621295331e-10 401895.540655962 -692779.586087855;-7.5e-05 5.1836631089363e-10 421320.185072211 -681140.907433425]  x3=[-0.000375 -1.05774996057314e-11 2516.12263919182 -3470.3824636051;-0.0003 -1.09417416631419e-11 2613.22665570726 -3397.863329624;-0.000225 -1.1297237059681e-11 2708.24169881783 -3322.62799568625;-0.00015 -1.16437016177682e-11 2801.09181495185 -3244.73660376666;-7.5e-05 -1.19808583789368e-11 2891.70278114715 -3164.25141905215]  x4=[-0.000375 1.77268678848373e-11 -263.637973265411 -2074.49907539812;-0.0003 1.81274022870555e-11 -204.885257542124 -2081.12319463842;-0.000225 1.8513445921244e-11 -145.968759678808 -2086.08369583918;-0.00015 1.88846901900283e-11 -86.9355766224015 -2089.37661365163;-7.5e-05 1.92408383264202e-11 -27.8328985962019 -2090.99931576767]  x5=0.000339324940197445  V1=ones(3,3)  V2=ones(3,3)  I1=ones(3,3)  I2=ones(3,3)  nHarmo=1  Measurements=None  Decoupling=off  VsMag0=[ 1 1 1]  VrMag0=[ 1 1 1]  VsAngle0=[0 -120 120]  VrAngle0=[0 -120 120]  IsMag0=[ 1 1 1]  IrMag0=[ 1 1 1]  IsAngle0=[0 -120 120]  IrAngle0=[0 -120 120]
      settings: AttributesFormatString=\n  LibrarySourceBlock=sps_lib/Power Grid Elements/Distributed Parameters Line
  Regulateurs6 : Subsystem
  Regulateurs7 : Subsystem
  "MIC7a " : PMIOPort  Side=Left
  MIC7b : PMIOPort  Port=2  Side=Left
  MIC7c : PMIOPort  Port=3  Side=Left
  QUE7a : PMIOPort  Port=4  Side=Left
  QUE7b : PMIOPort  Port=5  Side=Left
  QUE7c : PMIOPort  Port=6  Side=Left
  wires:
  Regulateurs6/1(Pm) -> "B_6 CHU-5600 MVA "/1
  Regulateurs6/2(Vf) -> "B_6 CHU-5600 MVA "/2
  "B_6 CHU-5600 MVA "/1 -> Regulateurs6/1(m)
  Regulateurs7/1(Pm) -> B_7 MAN 5000 MVA/1
  Regulateurs7/2(Vf) -> B_7 MAN 5000 MVA/2
  B_7 MAN 5000 MVA/1 -> Regulateurs7/1(m)
  connections:
  "Cs PER "/RConn3 -- MIC-LTD 409 km/LConn3
  "Cs PER "/RConn2 -- MIC-LTD 409 km/LConn2
  "Cs PER "/RConn1 -- MIC-LTD 409 km/LConn1
  Cs BER/RConn3 -- MAN-LEV 3*379km/LConn3
  Cs BER/RConn2 -- MAN-LEV 3*379km/LConn2
  Cs BER/RConn1 -- MAN-LEV 3*379km/LConn1
  Cs ARNS2/RConn3 -- ARN-MAN 2*169km/LConn3
  Cs ARNS2/RConn2 -- ARN-MAN 2*169km/LConn2
  Cs ARNS2/RConn1 -- ARN-MAN 2*169km/LConn1
  CHU-ARN 3*450km/RConn3 -- "Cs MTG+ARNN "/LConn3
  CHU-ARN 3*450km/RConn2 -- "Cs MTG+ARNN "/LConn2
  CHU-ARN 3*450km/RConn1 -- "Cs MTG+ARNN "/LConn1
  Load Flow Bus2/LConn1 -- 5600 MVA 13.8 kV/735 kV1/RConn3 -- CHU-ARN 3*450km/LConn3 -- CHU 330 Mvar/LConn3
  5600 MVA 13.8 kV/735 kV1/RConn2 -- CHU-ARN 3*450km/LConn2 -- CHU 330 Mvar/LConn2
  5600 MVA 13.8 kV/735 kV1/RConn1 -- CHU-ARN 3*450km/LConn1 -- CHU 330 Mvar/LConn1
  "B_6 CHU-5600 MVA "/RConn3 -- Load Flow Bus1/LConn1 -- 5600 MVA 13.8 kV/735 kV1/LConn3 -- 280 MW/LConn3
  5600 MVA 13.8 kV/735 kV1/LConn2 -- "B_6 CHU-5600 MVA "/RConn2 -- 280 MW/LConn2
  5600 MVA 13.8 kV/735 kV1/LConn1 -- "B_6 CHU-5600 MVA "/RConn1 -- 280 MW/LConn1
  "Cs ARNS1 "/RConn1 -- ARN-MIC 180km/LConn1
  "Cs ARNS1 "/RConn2 -- ARN-MIC 180km/LConn2
  "Cs ARNS1 "/RConn3 -- ARN-MIC 180km/LConn3
  "Cs PER "/LConn3 -- Load Flow Bus6/LConn1 -- MIC7c/RConn1 -- MIC-MAN 60 km/LConn3 -- ARN-MIC 180km/RConn3
  "Cs PER "/LConn2 -- MIC7b/RConn1 -- ARN-MIC 180km/RConn2 -- MIC-MAN 60 km/LConn2
  "Cs PER "/LConn1 -- "MIC7a "/RConn1 -- ARN-MIC 180km/RConn1 -- MIC-MAN 60 km/LConn1
  ARN-MAN 2*169km/RConn1 -- MAN7/LConn1
  ARN-MAN 2*169km/RConn2 -- MAN7/LConn2
  ARN-MAN 2*169km/RConn3 -- MAN7/LConn3
  Cs BER/LConn1 -- 5000 MVA 13.8 kV/735 kV2/RConn1 -- MIC-MAN 60 km/RConn1 -- MAN-MIC 1650 Mvar/LConn1 -- MAN7/RConn1
  Cs BER/LConn2 -- 5000 MVA 13.8 kV/735 kV2/RConn2 -- MIC-MAN 60 km/RConn2 -- MAN-MIC 1650 Mvar/LConn2 -- MAN7/RConn2
  Cs BER/LConn3 -- Load Flow Bus5/LConn1 -- 5000 MVA 13.8 kV/735 kV2/RConn3 -- MIC-MAN 60 km/RConn3 -- MAN-MIC 1650 Mvar/LConn3 -- MAN7/RConn3
  B_7 MAN 5000 MVA/RConn1 -- 5000 MVA 13.8 kV/735 kV2/LConn1 -- 250 MW/LConn1
  B_7 MAN 5000 MVA/RConn2 -- 5000 MVA 13.8 kV/735 kV2/LConn2 -- 250 MW/LConn2
  B_7 MAN 5000 MVA/RConn3 -- 5000 MVA 13.8 kV/735 kV2/LConn3 -- Load Flow Bus3/LConn1 -- 250 MW/LConn3
  MIC-LTD 409 km/RConn2 -- MAN-LEV 3*379km/RConn2 -- QUE7b/RConn1
  Cs ARNS2/LConn1 -- ARN 990 Mvar/LConn1 -- "Cs MTG+ARNN "/RConn1 -- "Cs ARNS1 "/LConn1
  Cs ARNS2/LConn2 -- ARN 990 Mvar/LConn2 -- "Cs MTG+ARNN "/RConn2 -- "Cs ARNS1 "/LConn2
  Cs ARNS2/LConn3 -- Load Flow Bus4/LConn1 -- "Cs ARNS1 "/LConn3 -- ARN 990 Mvar/LConn3 -- "Cs MTG+ARNN "/RConn3
  MIC-LTD 409 km/RConn1 -- QUE7a/RConn1 -- MAN-LEV 3*379km/RConn1
  MIC-LTD 409 km/RConn3 -- QUE7c/RConn1 -- MAN-LEV 3*379km/RConn3
